simulink model "Guidance"  (R2016b)
settings: Solver=VariableStepAuto  StartTime=0.0  StopTime=10.0  RelTol=1e-3
values from neighbouring files (symbols this model uses):
  direction_vm = -180 * Deg2Rad    (= -3.14159265359)    [Initialize.m]
  direction_vt = 0    [Initialize.m]
  Vm = 850    [Initialize.m]
  Vt = 300    [Initialize.m]
  xm0 = 5000    [Initialize.m]
  xt0 = 0    [Initialize.m]
  ym0 = 5000    [Initialize.m]
  yt0 = 0    [Initialize.m]
settings Model: Creator=SH  LastModifiedBy=SH

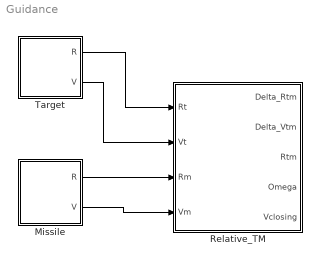
== system Guidance ==
  Missile : Subsystem
  Relative_TM : Subsystem
  Target : Subsystem
  wires:
  Target/1(R) -> Relative_TM/1(Rt)
  Target/2(V) -> Relative_TM/2(Vt)
  Missile/1(R) -> Relative_TM/3(Rm)
  Missile/2(V) -> Relative_TM/4(Vm)

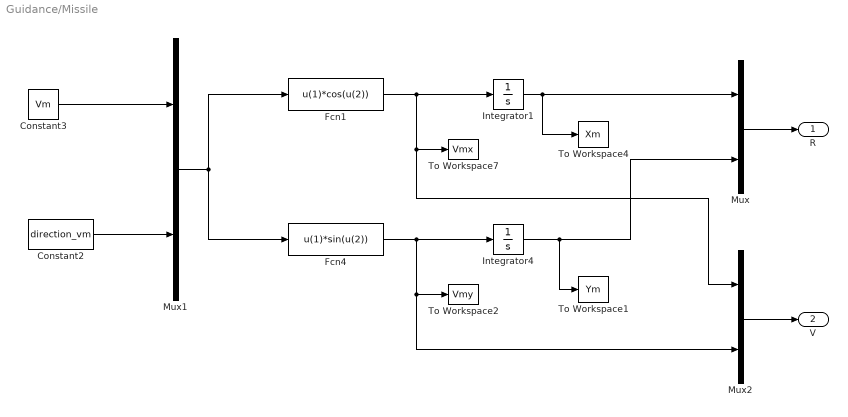
== system Guidance/Missile ==
  Constant2 : Constant  Value=direction_vm
  Constant3 : Constant  Value=Vm
  Fcn1 : Fcn  Expr=u(1)*cos(u(2))
  Fcn4 : Fcn  Expr=u(1)*sin(u(2))
  Integrator1 : Integrator  InitialCondition=xm0
  Integrator4 : Integrator  InitialCondition=ym0
  Mux : Mux  Inputs=2
  Mux1 : Mux  Inputs=2
  Mux2 : Mux  Inputs=2
  To Workspace1 : ToWorkspace  VariableName=Ym  SampleTime=-1
  To Workspace2 : ToWorkspace  VariableName=Vmy  SampleTime=-1
  To Workspace4 : ToWorkspace  VariableName=Xm  SampleTime=-1
  To Workspace7 : ToWorkspace  VariableName=Vmx  SampleTime=-1
  R : Outport
  V : Outport  Port=2
  wires:
  Mux/1 -> R/1
  Integrator1/1 -> Mux/1, To Workspace4/1
  Integrator4/1 -> Mux/2, To Workspace1/1
  Fcn4/1 -> Integrator4/1, Mux2/2, To Workspace2/1
  Mux1/1 -> Fcn1/1, Fcn4/1
  Fcn1/1 -> Integrator1/1, Mux2/1, To Workspace7/1
  Constant2/1 -> Mux1/2
  Constant3/1 -> Mux1/1
  Mux2/1 -> V/1

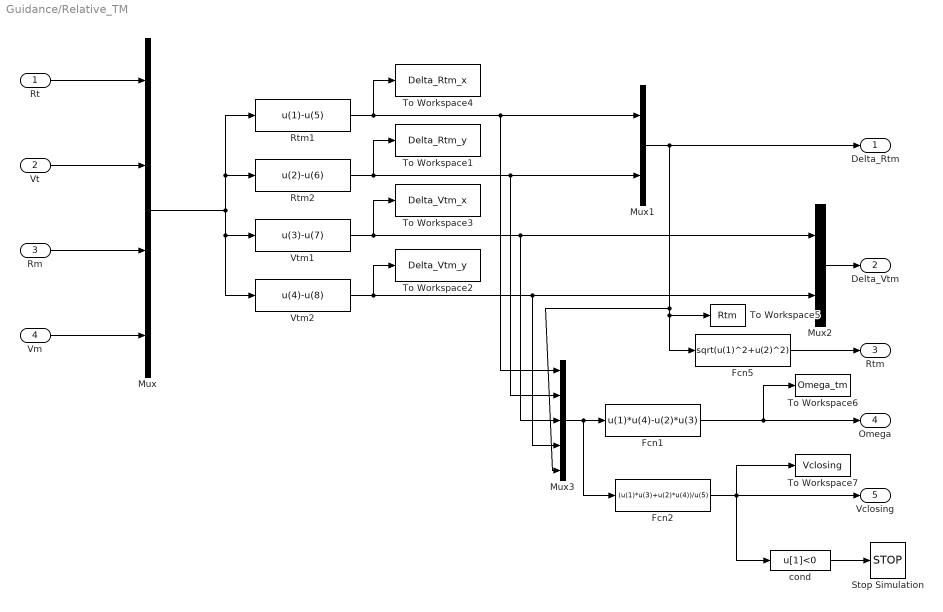
== system Guidance/Relative_TM ==
  Rt : Inport
  Vt : Inport  Port=2
  Rm : Inport  Port=3
  Vm : Inport  Port=4
  Fcn1 : Fcn  Expr=u(1)*u(4)-u(2)*u(3)
  Fcn2 : Fcn  Expr=(u(1)*u(3)+u(2)*u(4))/u(5)
  Fcn5 : Fcn  Expr=sqrt(u(1)^2+u(2)^2)
  Mux : Mux
  Mux1 : Mux  Inputs=2
  Mux2 : Mux  Inputs=2
  Mux3 : Mux  Inputs=5
  Rtm1 : Fcn  Expr=u(1)-u(5)
  Rtm2 : Fcn  Expr=u(2)-u(6)
  Stop Simulation : Stop
  To Workspace1 : ToWorkspace  VariableName=Delta_Rtm_y  SampleTime=-1
  To Workspace2 : ToWorkspace  VariableName=Delta_Vtm_y  SampleTime=-1
  To Workspace3 : ToWorkspace  VariableName=Delta_Vtm_x  SampleTime=-1
  To Workspace4 : ToWorkspace  VariableName=Delta_Rtm_x  SampleTime=-1
  To Workspace5 : ToWorkspace  VariableName=Rtm  SampleTime=-1
  To Workspace6 : ToWorkspace  VariableName=Omega_tm  SampleTime=-1
  To Workspace7 : ToWorkspace  VariableName=Vclosing  SampleTime=-1
  Vtm1 : Fcn  Expr=u(3)-u(7)
  Vtm2 : Fcn  Expr=u(4)-u(8)
  cond : Fcn  Expr=u[1]<0
  Delta_Rtm : Outport
  Delta_Vtm : Outport  Port=2
  Rtm : Outport  Port=3
  Omega : Outport  Port=4
  Vclosing : Outport  Port=5
  wires:
  Vm/1 -> Mux/4
  Rm/1 -> Mux/3
  Vt/1 -> Mux/2
  Rt/1 -> Mux/1
  Mux/1 -> Vtm2/1, Vtm1/1, Rtm1/1, Rtm2/1
  Rtm1/1 -> Mux3/1, Mux1/1, To Workspace4/1
  Rtm2/1 -> Mux3/2, Mux1/2, To Workspace1/1
  Vtm1/1 -> Mux3/3, Mux2/1, To Workspace3/1
  Vtm2/1 -> Mux3/4, Mux2/2, To Workspace2/1
  Mux1/1 -> Mux3/5, Fcn5/1, To Workspace5/1, Delta_Rtm/1
  Mux2/1 -> Delta_Vtm/1
  Fcn5/1 -> Rtm/1
  Mux3/1 -> Fcn2/1, Fcn1/1
  Fcn1/1 -> To Workspace6/1, Omega/1
  Fcn2/1 -> To Workspace7/1, cond/1, Vclosing/1
  cond/1 -> Stop Simulation/1

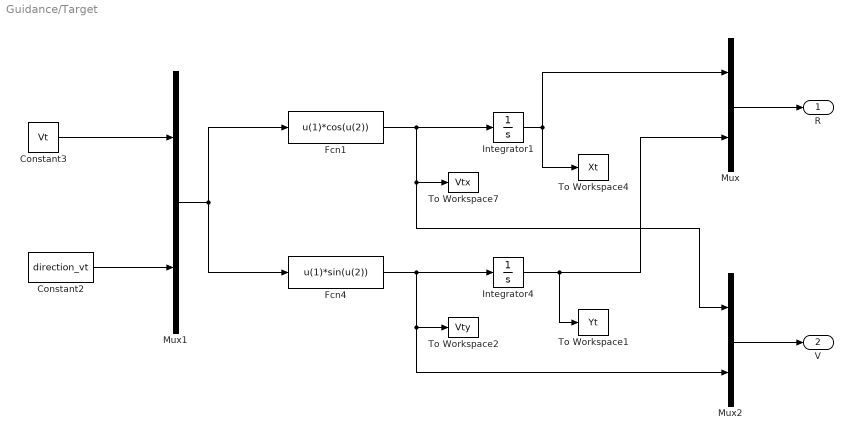
== system Guidance/Target ==
  Constant2 : Constant  Value=direction_vt
  Constant3 : Constant  Value=Vt
  Fcn1 : Fcn  Expr=u(1)*cos(u(2))
  Fcn4 : Fcn  Expr=u(1)*sin(u(2))
  Integrator1 : Integrator  InitialCondition=xt0
  Integrator4 : Integrator  InitialCondition=yt0
  Mux : Mux  Inputs=2
  Mux1 : Mux  Inputs=2
  Mux2 : Mux  Inputs=2
  To Workspace1 : ToWorkspace  VariableName=Yt  SampleTime=-1
  To Workspace2 : ToWorkspace  VariableName=Vty  SampleTime=-1
  To Workspace4 : ToWorkspace  VariableName=Xt  SampleTime=-1
  To Workspace7 : ToWorkspace  VariableName=Vtx  SampleTime=-1
  R : Outport
  V : Outport  Port=2
  wires:
  Constant3/1 -> Mux1/1
  Constant2/1 -> Mux1/2
  Fcn1/1 -> Mux2/1, To Workspace7/1, Integrator1/1
  Mux1/1 -> Fcn4/1, Fcn1/1
  Fcn4/1 -> Mux2/2, To Workspace2/1, Integrator4/1
  Integrator4/1 -> To Workspace1/1, Mux/2
  Integrator1/1 -> To Workspace4/1, Mux/1
  Mux/1 -> R/1
  Mux2/1 -> V/1
